simulink model "highgain_with_data_record_param_lowpass"  (R2021b)
settings: Solver=FixedStepDiscrete  StartTime=0.0  StopTime=10.0  RelTol=1e-3
values from neighbouring files (symbols this model uses):
  DEG2RAD = 0.0174533    [init.m]
  MAX_ATTI_INTEGRAL_SAT_LOWER = -1    [init.m]
  MAX_ATTI_INTEGRAL_SAT_UPPPER = 1    [init.m]
  MAX_ATTI_ROLLPITCH_CONTROL_COMMAND = 220 * DEG2RAD    (= 3.839726)    [init.m]
  MAX_ATTI_YAW_CONTROL_COMMAND = 200 * DEG2RAD    (= 3.49066)    [init.m]
  MAX_CONTROL_ANGLE_PITCH = 35    [init.m]
  MAX_CONTROL_ANGLE_RATE_Y = 200    [init.m]
  MAX_CONTROL_ANGLE_ROLL = 35    [init.m]
  MC_ROLL_P = Pixhawk_CSC.Parameter( {single(1), 'MC_ROLL_P'})    [init.m]
  MC_ROLLRATE_D = Pixhawk_CSC.Parameter( {single(1), 'MC_ROLLRATE_D'})    [init.m]
  MC_ROLLRATE_I = Pixhawk_CSC.Parameter( {single(1), 'MC_ROLLRATE_I'})    [init.m]
  MC_ROLLRATE_P = Pixhawk_CSC.Parameter( {single(1), 'MC_ROLLRATE_P'})    [init.m]
  THR_HOVER = 0.609    [init.m]
undefined symbols (not defined in the file or in its folder): DiscIntNeverNeededParam, RGBLED_COLOR_ENUM, RGBLED_MODE_ENUM
libraries: simulink x7, pixhawk_slib_sensors_actuators x5, pixhawk_slib_uORB_RW x4
settings Model: Creator=wsh  LastModifiedBy=jimdi
settings SolverCC: AlgebraicLoopSolver=TrustRegion
settings DataIOCC: ReturnWorkspaceOutputs=off
settings OptimizationCC: DefaultParameterBehavior=Inlined  MaxStackSize=64  EfficientTunableParamExpr=on
settings DebuggingCC: ParameterTunabilityLossMsg=error  SFMachineParentedDataDiag=warning  ArithmeticOperatorsInVariantConditions=warning
settings HardwareCC: ProdBitPerPointer=32  ProdBitPerSizeT=32  ProdBitPerPtrDiffT=32  ProdLargestAtomicInteger=Long  ProdLargestAtomicFloat=Double  ProdWordSize=32  ProdHWDeviceType=ARM Compatible->ARM Cortex
settings SFSimCC: SimUseLocalCustomCode=off  MATLABDynamicMemAlloc=off  CustomCodeUndefinedFunction=UseInterfaceOnly
settings RTWCC: Description=Embedded Coder  SystemTargetFile=ert.tlc  HardwareBoard=Pixhawk PX4  TLCOptions="-aInlineSetEventsForThisBaseRateFcn=TLC_FALSE -aSuppressMultiTaskScheduler=TLC_FALSE  -aRateBasedStepFcn=0"  TemplateMakefile=ert_default_tmf  GenerateReport=on  RTWUseLocalCustomCode=off  Toolchain=Pixhawk Toolchain  IncludeHyperlinkInReport=on  LaunchReport=on  GenerateTraceInfo=on  GenerateTraceReport=on  GenerateTraceReportSl=on  GenerateTraceReportSf=on  GenerateTraceReportEml=on
settings CodeAppCC: ForceParamTrailComments=on  IgnoreCustomStorageClasses=off  OperatorAnnotations=on  SimulinkDataObjDesc=on  SFDataObjDesc=on  MATLABFcnDesc=on  InsertBlockDesc=on  StateflowObjectComments=on  MATLABSourceComments=on
settings ERTTargetCC: MultiwordLength=2048  ERTCustomFileTemplate=PX4_codertarget_file_process.tlc

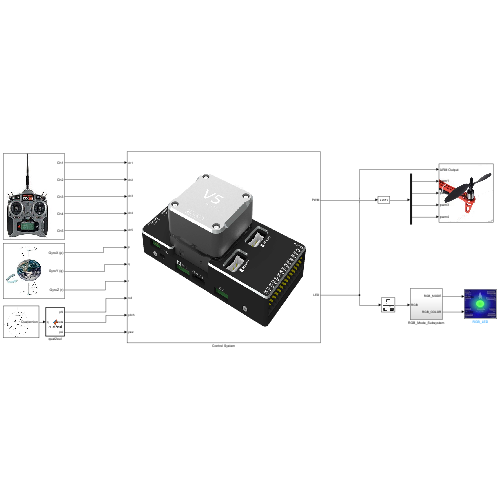
[thumbnail: Simulink's stored preview of the top-level diagram]
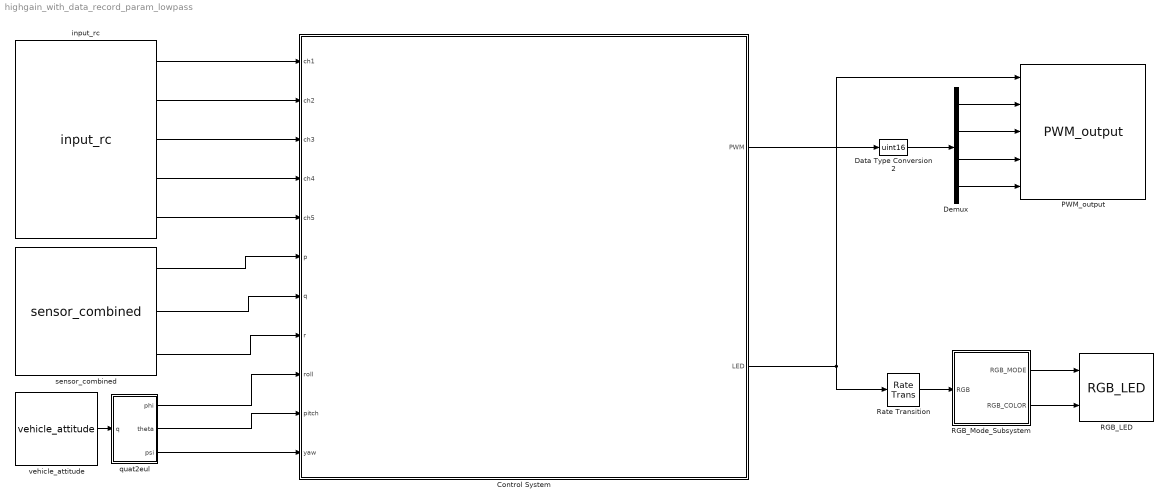
== system highgain_with_data_record_param_lowpass ==
  Control System : Subsystem
      mask Display: image('icon\pixhawk.png');
  Data Type Conversion2 : DataTypeConversion  OutDataTypeStr=uint16
  Demux : Demux
  PWM_output : pixhawk_slib_sensors_actuators/PWM_output  Description=|  pub_outputs=on  pwm_rate=400Hz  show_pwm1=on  show_pwm5=off  show_pwm2=on  show_pwm6=off  show_pwm3=on  show_pwm7=off  show_pwm4=on  show_pwm8=off
      | This block allows the user to send the appropriate PWM signals out to the PX4 outputs.  
      | These are usually connected to the ESCs which control the motor speeds. 
      | In order for the flight control to arm (enable) the output from the software side, the ARM Output input must be held high (boolean TRUE).  
      | Only then will the PWM values be sent out the PX4 hardware ports.  
      | This is usually a function of the RC Tx in combination with other flight modes programmed in the Simulink model by the user.  
      | The block has 8 available ports (data type uint16) which can be selectively chosen.  
      | These correspond to the 8 PWM output ports on the px4fmu hardware.
      settings: SourceProductName=Pixhawk Target Blocks
  RGB_LED : pixhawk_slib_sensors_actuators/RGB_LED
      settings: SourceProductName=Pixhawk Target Blocks
  RGB_Mode_Subsystem : Subsystem
  Rate Transition : RateTransition  OutPortSampleTime=1
  input_rc : pixhawk_slib_sensors_actuators/input_rc  Description=|  sampletime=0.004  channel1=on  channel2=on  channel3=on  channel4=on  channel5=on  channel6=off  channel7=off  channel8=off  channel9=off  channel10=off  channel11=off  channel12=off  channel13=off  channel14=off  channel15=off  channel16=off  channel17=off  channel18=off  ch_count=off  rssi=off  rc_failsafe=off  rc_lost=off  rc_inputsource=off
      | RC Input Block
      | 
      | This block provides user input control to the model.
      | It uses the input_rc uORB topic.
      | 
      | The user has the ability to choose which channels are available as outputs from this block and also some optional outputs. These include 
      | Channels 1 through 18
      | double data type indicating the PWM value from the controller 
      | measured pulse widths for each of the supported channels 
      | Channel Count 
      | uint32 data type of the number of channels which are detector by the PX4 
      | RC Failsafe 
      | boolean data types indicating that the RC Tx is sending the FailSafe signal (if equipped and properly setup) 
      | explicit failsafe flag: true on TX failure or TX out of range , false otherwise. 
      | Only the true state is reliable, as there are some (PPM) receivers on the market going into failsafe without telling us explicitly. 
      | RC Input Source 
      | Enumeration data type indicating which source the RC input is from. 
      | Valid values are found in the ENUM file: RC_INPUT_SOURCE_ENUM.m 
      |           Enumeration members for class 'RC_INPUT_SOURCE_ENUM':
      |           RCINPUT_SOURCE_UNKNOWN         (0)
      |           RCINPUT_SOURCE_PX4FMU_PPM      (1)
      |           RCINPUT_SOURCE_PX4IO_PPM       (2)
      |           RCINPUT_SOURCE_PX4IO_SPEKTRUM  (3)
      |           RCINPUT_SOURCE_PX4IO_SBUS      (4)
      |           RCINPUT_SOURCE_PX4IO_ST24      (5)
      |           RCINPUT_SOURCE_MAVLINK         (6)
      |           RCINPUT_SOURCE_QURT            (7)
      |           RCINPUT_SOURCE_PX4FMU_SPEKTRUM (8)
      |           RCINPUT_SOURCE_PX4FMU_SBUS     (9)
      |           RCINPUT_SOURCE_PX4FMU_ST24     (10)
      |           RCINPUT_SOURCE_PX4FMU_SUMD     (11)
      |           RCINPUT_SOURCE_PX4FMU_DSM      (12)
      |           RCINPUT_SOURCE_PX4IO_SUMD      (13)
      | 
      | RSSI - Receive signal strength index 
      | receive signal strength indicator (RSSI): < 0: Undefined, 0: no signal, 255: full reception 
      | RC Lost Connection 
      | boolean data type indicating RC receiver connection status 
      | True, if no frame has arrived in the expected time, false otherwise. 
      | True usally means that the receiver has been disconnected, but can also indicate a radio link loss on "stupid" systems. 
      | Will remain false, if a RX with failsafe option continues to transmit frames after a link loss. 
      |   
      | Sample Model: px4demo_input_rc.slx
      settings: SourceProductName=Pixhawk Target Blocks
  quat2eul : MATLAB Function  TreatAsAtomicUnit=on
  sensor_combined : pixhawk_slib_sensors_actuators/sensor_combined  Description=|  sampletime=0.004  show_mag=off  show_acc=off  show_gyro=on  show_baro=off  show_ts=off
      | Sensor Combined Block
      | 
      | This block enables access to the various sensors available on the px4fmu-v2 hardware.  
      | The user can use these signals in the Simulink control model.  
      | The sample time needs to be provided in the mask dialog.  
      | Optional output ports can also be selected.  
      | Refer to the sample model: px4demo_attitude_control.slx
      | 
      | Signal definitions: 
      | Magnetometer (x,y,z) - single values – Magnetic field in NED body frame, in Gauss 
      | Accelerometer (x,y,z) - single values – Acceleration in NED body frame, in m/s^2 
      | Gyroscope (p,q,r) - single values – Angular velocity in radians per second 
      | Barometer (Altitude) - single value – Barometric pressure, already temperature compensated (millibars) 
      | RunTime (timestamp) - double value – Timestamp in microseconds since boot, from gyro 
      |   
      | The sensor_combined block needs to have the px4io service running on the PX4 hardware in order to get valid signal values.
      settings: SourceProductName=Pixhawk Target Blocks
  vehicle_attitude : pixhawk_slib_sensors_actuators/vehicle_attitude  Description=|  sampletime=0.004  show_r=off  show_p=off  show_y=off  show_q=on  show_ts=off
      | This block gives access to the running service that calculates the vehicle’s attitude.  A uORB topic (vehicle_attitude (attitude measurements)) publisher MUST be running in order for this block to provide valid signal values.  The available ones as of v1.3 are: 
      | attitude_estimator_ekf – EKF-Extended Kalman Filter for attitude estimation 
      | attitude_estimator_so3 – SO(3)-attitude estimation by using accelerometer, gyroscopes and magnetometer 
      | One of these MUST be running on the px4fmu in order for this block to return valid values.  Refer to the sample model: px4demo_attitude_control.slx. Attitude in NED (North-East-Down) body frame in SI units. 
      | Signal definitions: 
      | Roll – single value, Roll angle (rad, Tait-Bryan, NED) 
      | Pitch – single value, Pitch angle (rad, Tait-Bryan, NED) 
      | Yaw – single value, Yaw angle (rad, Tait-Bryan, NED) 
      | Quaternion (NED) – single(4) values (optional based on the uORB publisher)
      settings: SourceProductName=Pixhawk Target Blocks
  wires:
  sensor_combined/1 -> Control System/6(p)
  sensor_combined/3 -> Control System/8(r)
  quat2eul/1(phi) -> Control System/9(roll)
  quat2eul/2(theta) -> Control System/10(pitch)
  sensor_combined/2 -> Control System/7(q)
  Control System/1(PWM) -> Data Type Conversion2/1
  Data Type Conversion2/1 -> Demux/1
  Demux/1 -> PWM_output/2
  Demux/2 -> PWM_output/3
  Demux/3 -> PWM_output/4
  Demux/4 -> PWM_output/5
  input_rc/1 -> Control System/1(ch1)
  input_rc/2 -> Control System/2(ch2)
  input_rc/3 -> Control System/3(ch3)
  input_rc/4 -> Control System/4(ch4)
  input_rc/5 -> Control System/5(ch5)
  RGB_Mode_Subsystem/2(RGB_COLOR) -> RGB_LED/2
  Rate Transition/1 -> RGB_Mode_Subsystem/1(RGB)
  RGB_Mode_Subsystem/1(RGB_MODE) -> RGB_LED/1
  Control System/2(LED) -> Rate Transition/1, PWM_output/1
  vehicle_attitude/1 -> quat2eul/1(q)
  quat2eul/3(psi) -> Control System/11(yaw)

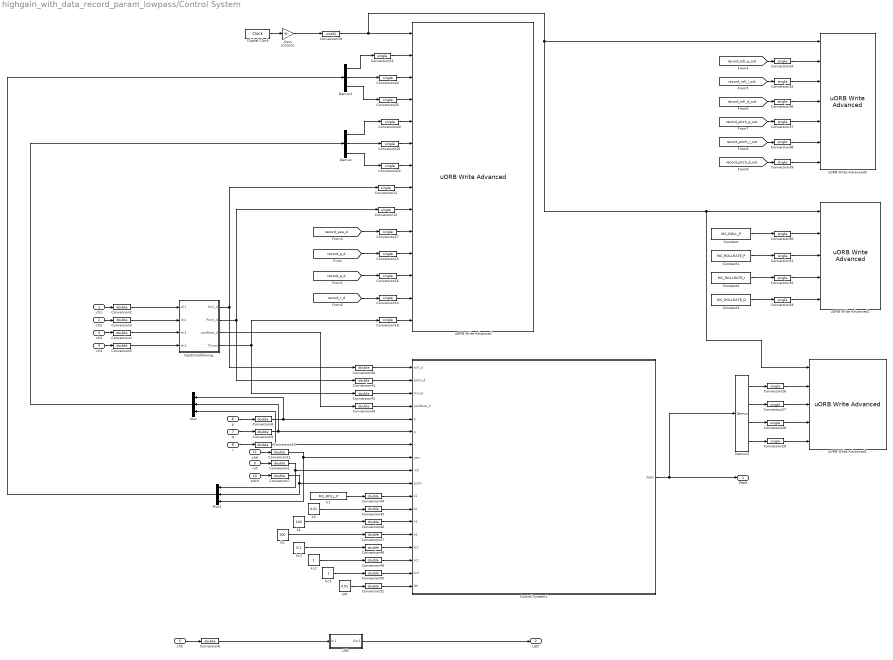
== system highgain_with_data_record_param_lowpass/Control System ==
  ch1 : Inport  OutDataTypeStr=uint16  PortDimensions=1
  ch2 : Inport  Port=2  OutDataTypeStr=uint16  PortDimensions=1
  ch3 : Inport  Port=3  OutDataTypeStr=uint16  PortDimensions=1
  ch4 : Inport  Port=4  OutDataTypeStr=uint16  PortDimensions=1
  ch5 : Inport  Port=5  OutDataTypeStr=uint16  PortDimensions=1  Interpolate=off
  p : Inport  Port=6  PortDimensions=1
  q : Inport  Port=7  PortDimensions=1
  r : Inport  Port=8  PortDimensions=1
  roll : Inport  Port=9  PortDimensions=1
  pitch : Inport  Port=10  PortDimensions=1
  yaw : Inport  Port=11  PortDimensions=1
  Constant : Constant  Value=MC_ROLL_P
  Constant1 : Constant  Value=MC_ROLLRATE_P
  Constant2 : Constant  Value=MC_ROLLRATE_I
  Constant3 : Constant  Value=MC_ROLLRATE_D
  Control System1 : Subsystem
      mask Display: image('test_bench.png'); % 使用工具条上的 "编辑图像" 进行更改。
  Conversion{1..11,40..51} (23 alike) : DataTypeConversion  OutDataTypeStr=double
  Conversion{12..18,20..39} (27 alike) : DataTypeConversion  OutDataTypeStr=single
  Conversion19 : DataTypeConversion  OutDataTypeStr=uint32
  Demux : Demux  Outputs=3
  Demux1 : Demux  Outputs=3
  Demux2 : Demux
  Digital Clock : DigitalClock  SampleTime=-1
  Gain : Gain  Gain=1000000
  InputConditioning : Subsystem
  "LED " : Subsystem
  Mux : Mux  Inputs=3
  Mux1 : Mux  Inputs=3
  h1 : Constant  Value=100
  h2 : Constant  Value=100
  k1 : Constant  Value=MC_ROLL_P
  k2 : Constant  Value=0.01
  kM : Constant  Value=0.01
  kc1 : Constant  Value=0.1
  kc2 : Constant
  kc3 : Constant
  uORB Write Advanced{,1..3} (4 alike) : pixhawk_slib_uORB_RW/uORB Write Advanced  Ts=0  uORB_AdvtQueue=on  uORB_FieldEnabledArr="0  0  0  1  0  0  0  0  0  0  0"  uORB_Topic_str=0  uORB_Struct_DT="[1  1  1  1  1]"  BlockInputCount=5  uORB_StructParams="[\"voltage_v\",\"voltage_filtered_v\",\"current_a\",\"current_filtered_a\",\"remaining\"]"  uORB_PortSizes="[1  1  1  1]"  MsgSizeOf=0  MW_update=true
      settings: SourceProductName=Pixhawk Target Blocks
  PWM : Outport  VectorParamsAs1DForOutWhenUnconnected=off
  LED : Outport  Port=2  PortDimensions=1  VectorParamsAs1DForOutWhenUnconnected=off
  wires:
  kc1/1 -> Conversion48/1
  Conversion9/1 -> Mux/2, Control System1/6(q)
  p/1 -> Conversion8/1
  "LED "/1(Out1) -> LED/1
  kM/1 -> Conversion51/1
  Conversion11/1 -> Mux1/3, Control System1/8(yaw)
  Control System1/1(PWM) -> Demux2/1, PWM/1
  Conversion4/1 -> InputConditioning/3(ch3)
  h2/1 -> Conversion47/1
  ch1/1 -> Conversion2/1
  h1/1 -> Conversion46/1
  ch4/1 -> Conversion5/1
  InputConditioning/4(Thrust) -> Conversion18/1, Conversion42/1
  Conversion2/1 -> InputConditioning/1("ch1 ")
  InputConditioning/3(yawRate_d) -> Conversion43/1
  Conversion1/1 -> Mux1/1, Control System1/9(roll)
  Conversion7/1 -> Mux1/2, Control System1/10(pitch)
  yaw/1 -> Conversion11/1
  kc3/1 -> Conversion50/1
  kc2/1 -> Conversion49/1
  Conversion8/1 -> Control System1/5(p), Mux/1
  InputConditioning/1(Roll_d) -> Conversion40/1, Conversion12/1
  Conversion10/1 -> Mux/3, Control System1/7(r)
  roll/1 -> Conversion1/1
  InputConditioning/2(Pitch_d) -> Conversion41/1, Conversion13/1
  k2/1 -> Conversion45/1
  Conversion3/1 -> InputConditioning/2(ch2)
  pitch/1 -> Conversion7/1
  r/1 -> Conversion10/1
  Conversion5/1 -> InputConditioning/4(ch4)
  Conversion6/1 -> "LED "/1(In1)
  ch2/1 -> Conversion3/1
  ch5/1 -> Conversion6/1
  ch3/1 -> Conversion4/1
  q/1 -> Conversion9/1
  Gain/1 -> Conversion19/1
  Conversion19/1 -> uORB Write Advanced2/1, uORB Write Advanced1/1, uORB Write Advanced3/1, uORB Write Advanced/1
  Digital Clock/1 -> Gain/1
  Conversion12/1 -> uORB Write Advanced/8
  Conversion13/1 -> uORB Write Advanced/9
  Mux/1 -> Demux/1
  Mux1/1 -> Demux1/1
  [record_p_d] -> Conversion15/1
  Conversion15/1 -> uORB Write Advanced/11
  Conversion16/1 -> uORB Write Advanced/12
  [record_q_d] -> Conversion16/1
  [record_r_d] -> Conversion14/1
  Conversion14/1 -> uORB Write Advanced/13
  [record_yaw_d] -> Conversion17/1
  Conversion17/1 -> uORB Write Advanced/10
  Conversion18/1 -> uORB Write Advanced/14
  Conversion20/1 -> uORB Write Advanced/5
  Conversion22/1 -> uORB Write Advanced/7
  Conversion21/1 -> uORB Write Advanced/6
  Demux/1 -> Conversion20/1
  Demux/2 -> Conversion21/1
  Demux/3 -> Conversion22/1
  Conversion25/1 -> uORB Write Advanced/4
  Conversion24/1 -> uORB Write Advanced/3
  Conversion23/1 -> uORB Write Advanced/2
  Demux1/1 -> Conversion23/1
  Demux1/2 -> Conversion24/1
  Demux1/3 -> Conversion25/1
  Conversion29/1 -> uORB Write Advanced1/5
  Conversion28/1 -> uORB Write Advanced1/4
  Conversion27/1 -> uORB Write Advanced1/3
  Conversion26/1 -> uORB Write Advanced1/2
  Demux2/1 -> Conversion26/1
  Demux2/2 -> Conversion27/1
  Demux2/3 -> Conversion28/1
  Demux2/4 -> Conversion29/1
  Conversion30/1 -> uORB Write Advanced2/2
  Conversion33/1 -> uORB Write Advanced2/5
  Conversion32/1 -> uORB Write Advanced2/4
  Conversion31/1 -> uORB Write Advanced2/3
  Constant/1 -> Conversion30/1
  Constant1/1 -> Conversion31/1
  Constant2/1 -> Conversion32/1
  Constant3/1 -> Conversion33/1
  Conversion34/1 -> uORB Write Advanced3/2
  [record_roll_p_out] -> Conversion34/1
  [record_roll_i_out] -> Conversion35/1
  Conversion35/1 -> uORB Write Advanced3/3
  Conversion36/1 -> uORB Write Advanced3/4
  [record_roll_d_out] -> Conversion36/1
  [record_pitch_p_out] -> Conversion37/1
  [record_pitch_i_out] -> Conversion38/1
  [record_pitch_d_out] -> Conversion39/1
  Conversion37/1 -> uORB Write Advanced3/5
  Conversion38/1 -> uORB Write Advanced3/6
  Conversion39/1 -> uORB Write Advanced3/7
  Conversion40/1 -> Control System1/1(roll_d)
  Conversion41/1 -> Control System1/2(pitch_d)
  Conversion42/1 -> Control System1/3(thrust)
  Conversion43/1 -> Control System1/4(yawRate_d)
  k1/1 -> Conversion44/1
  Conversion44/1 -> Control System1/11(k1)
  Conversion45/1 -> Control System1/12(k2)
  Conversion46/1 -> Control System1/13(h1)
  Conversion47/1 -> Control System1/14(h2)
  Conversion48/1 -> Control System1/15(kc1)
  Conversion49/1 -> Control System1/16(kc2)
  Conversion50/1 -> Control System1/17(kc3)
  Conversion51/1 -> Control System1/18(kM)

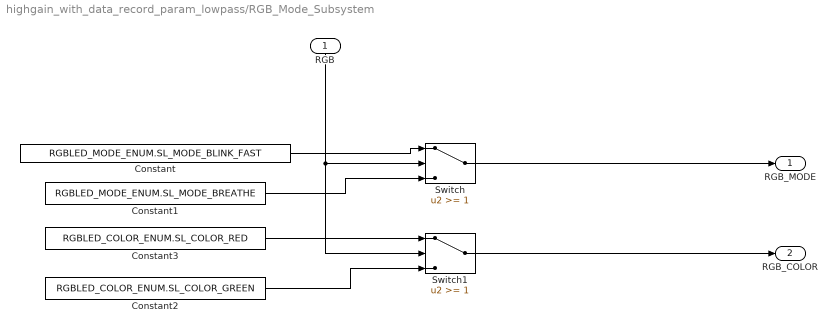
== system highgain_with_data_record_param_lowpass/RGB_Mode_Subsystem ==
  RGB : Inport
  Constant : Constant  Value=RGBLED_MODE_ENUM.SL_MODE_BLINK_FAST  OutDataTypeStr=Enum: RGBLED_MODE_ENUM
  Constant1 : Constant  Value=RGBLED_MODE_ENUM.SL_MODE_BREATHE  OutDataTypeStr=Enum: RGBLED_MODE_ENUM
  Constant2 : Constant  Value=RGBLED_COLOR_ENUM.SL_COLOR_GREEN  OutDataTypeStr=Enum: RGBLED_COLOR_ENUM
  Constant3 : Constant  Value=RGBLED_COLOR_ENUM.SL_COLOR_RED  OutDataTypeStr=Enum: RGBLED_COLOR_ENUM
  Switch : Switch  Threshold=1
  Switch1 : Switch  Threshold=1
  RGB_MODE : Outport  VectorParamsAs1DForOutWhenUnconnected=off
  RGB_COLOR : Outport  Port=2  VectorParamsAs1DForOutWhenUnconnected=off
  wires:
  RGB/1 -> Switch1/2, Switch/2
  Constant/1 -> Switch/1
  Constant1/1 -> Switch/3
  Switch/1 -> RGB_MODE/1
  Constant3/1 -> Switch1/1
  Constant2/1 -> Switch1/3
  Switch1/1 -> RGB_COLOR/1

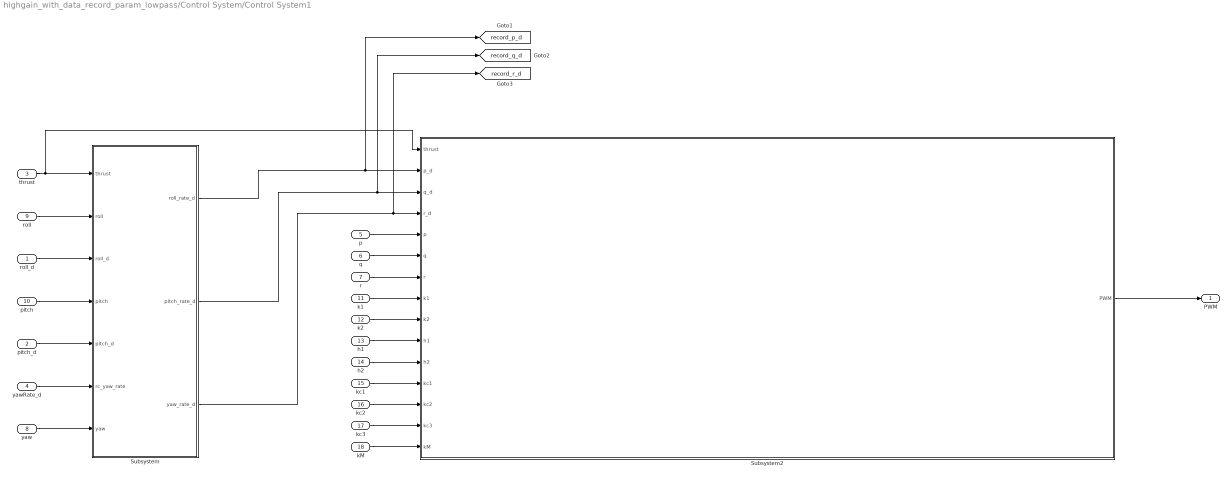
== system highgain_with_data_record_param_lowpass/Control System/Control System1 ==
  roll_d : Inport  PortDimensions=1
  pitch_d : Inport  Port=2  PortDimensions=1
  thrust : Inport  Port=3  PortDimensions=1
  yawRate_d : Inport  Port=4  PortDimensions=1
  p : Inport  Port=5  PortDimensions=1
  q : Inport  Port=6  PortDimensions=1
  r : Inport  Port=7  PortDimensions=1
  yaw : Inport  Port=8  PortDimensions=1
  roll : Inport  Port=9  PortDimensions=1
  pitch : Inport  Port=10  PortDimensions=1
  k1 : Inport  Port=11  PortDimensions=1
  k2 : Inport  Port=12  PortDimensions=1
  h1 : Inport  Port=13  PortDimensions=1
  h2 : Inport  Port=14  PortDimensions=1
  kc1 : Inport  Port=15  PortDimensions=1
  kc2 : Inport  Port=16  PortDimensions=1
  kc3 : Inport  Port=17  PortDimensions=1
  kM : Inport  Port=18  PortDimensions=1
  Subsystem : Subsystem
  Subsystem2 : Subsystem
      mask Display: image('angular_control_architecture.png'); % 使用工具条上的 "编辑图像" 进行更改。
  PWM : Outport  VectorParamsAs1DForOutWhenUnconnected=off
  tag scope: record_p_d=global, record_q_d=global, record_r_d=global
  wires:
  q/1 -> Subsystem2/6(q)
  r/1 -> Subsystem2/7(r)
  Subsystem2/1(PWM) -> PWM/1
  p/1 -> Subsystem2/5(p)
  k1/1 -> Subsystem2/8(k1)
  k2/1 -> Subsystem2/9(k2)
  h1/1 -> Subsystem2/10(h1)
  h2/1 -> Subsystem2/11(h2)
  kc1/1 -> Subsystem2/12(kc1)
  kc2/1 -> Subsystem2/13(kc2)
  kc3/1 -> Subsystem2/14(kc3)
  kM/1 -> Subsystem2/15(kM)
  thrust/1 -> Subsystem2/1(thrust), Subsystem/1(thrust)
  Subsystem/3(yaw_rate_d) -> [record_r_d], Subsystem2/4(r_d)
  Subsystem/2(pitch_rate_d) -> [record_q_d], Subsystem2/3(q_d)
  Subsystem/1(roll_rate_d) -> [record_p_d], Subsystem2/2(p_d)
  roll/1 -> Subsystem/2(roll)
  roll_d/1 -> Subsystem/3(roll_d)
  pitch/1 -> Subsystem/4(pitch)
  pitch_d/1 -> Subsystem/5(pitch_d)
  yawRate_d/1 -> Subsystem/6(rc_yaw_rate)
  yaw/1 -> Subsystem/7(yaw)

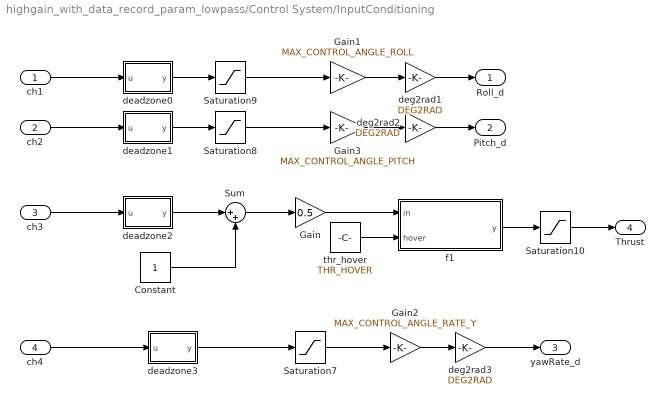
== system highgain_with_data_record_param_lowpass/Control System/InputConditioning ==
  "ch1 " : Inport
  ch2 : Inport  Port=2
  ch3 : Inport  Port=3
  ch4 : Inport  Port=4
  Constant : Constant
  Gain : Gain  Gain=0.5
  Gain1 : Gain  Gain=MAX_CONTROL_ANGLE_ROLL  OutDataTypeStr=Inherit: Inherit via back propagation
  Gain2 : Gain  Gain=MAX_CONTROL_ANGLE_RATE_Y
  Gain3 : Gain  Gain=MAX_CONTROL_ANGLE_PITCH  OutDataTypeStr=Inherit: Inherit via back propagation
  Saturation10 : Saturate  UpperLimit=1  LowerLimit=0
  Saturation7 : Saturate  UpperLimit=1  LowerLimit=-1
  Saturation8 : Saturate  UpperLimit=1  LowerLimit=-1
  Saturation9 : Saturate  UpperLimit=1  LowerLimit=-1
  Sum : Sum  Inputs=|++
  deadzone0 : MATLAB Function  TreatAsAtomicUnit=on
  deadzone1 : MATLAB Function  TreatAsAtomicUnit=on
  deadzone2 : MATLAB Function  TreatAsAtomicUnit=on
  deadzone3 : MATLAB Function  TreatAsAtomicUnit=on
  deg2rad1 : Gain  Gain=DEG2RAD
  deg2rad2 : Gain  Gain=DEG2RAD
  deg2rad3 : Gain  Gain=DEG2RAD
  f1 : MATLAB Function  TreatAsAtomicUnit=on
  "thr_hover " : Constant  Value=THR_HOVER
  Roll_d : Outport  VectorParamsAs1DForOutWhenUnconnected=off
  Pitch_d : Outport  Port=2  VectorParamsAs1DForOutWhenUnconnected=off
  yawRate_d : Outport  Port=3  VectorParamsAs1DForOutWhenUnconnected=off
  Thrust : Outport  Port=4  VectorParamsAs1DForOutWhenUnconnected=off
  wires:
  deadzone2/1(y) -> Sum/1
  ch3/1 -> deadzone2/1(u)
  deadzone1/1(y) -> Saturation8/1
  Saturation10/1 -> Thrust/1
  deadzone0/1(y) -> Saturation9/1
  "ch1 "/1 -> deadzone0/1(u)
  ch2/1 -> deadzone1/1(u)
  Saturation9/1 -> Gain1/1
  Saturation8/1 -> Gain3/1
  Gain3/1 -> deg2rad2/1
  Constant/1 -> Sum/2
  Sum/1 -> Gain/1
  Gain1/1 -> deg2rad1/1
  deg2rad1/1 -> Roll_d/1
  deg2rad2/1 -> Pitch_d/1
  Saturation7/1 -> Gain2/1
  deadzone3/1(y) -> Saturation7/1
  ch4/1 -> deadzone3/1(u)
  Gain2/1 -> deg2rad3/1
  deg2rad3/1 -> yawRate_d/1
  "thr_hover "/1 -> f1/2(hover)
  Gain/1 -> f1/1(in)
  f1/1(y) -> Saturation10/1

== system highgain_with_data_record_param_lowpass/Control System/LED  ==
  In1 : Inport
  Compare To Constant3 : simulink/Logic and Bit Operations/Compare To Constant  relop=>=  const=uint16(1500)  OutDataTypeStr=boolean
  Out1 : Outport  VectorParamsAs1DForOutWhenUnconnected=off
  wires:
  Compare To Constant3/1 -> Out1/1
  In1/1 -> Compare To Constant3/1

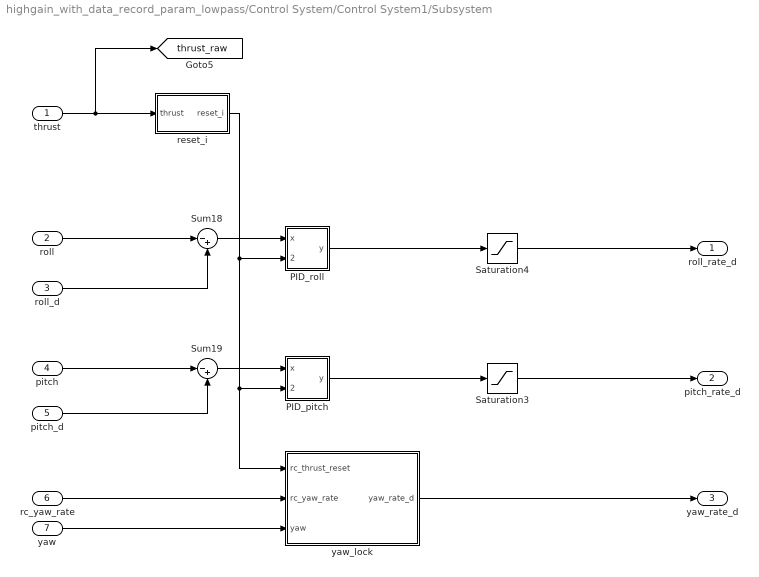
== system highgain_with_data_record_param_lowpass/Control System/Control System1/Subsystem ==
  thrust : Inport
  roll : Inport  Port=2
  roll_d : Inport  Port=3
  pitch : Inport  Port=4
  pitch_d : Inport  Port=5
  rc_yaw_rate : Inport  Port=6
  yaw : Inport  Port=7
  PID_pitch : Subsystem
  "PID_roll " : Subsystem
  Saturation3 : Saturate  UpperLimit=MAX_ATTI_ROLLPITCH_CONTROL_COMMAND  LowerLimit=-MAX_ATTI_ROLLPITCH_CONTROL_COMMAND
  Saturation4 : Saturate  UpperLimit=MAX_ATTI_ROLLPITCH_CONTROL_COMMAND  LowerLimit=-MAX_ATTI_ROLLPITCH_CONTROL_COMMAND
  Sum18 : Sum  Inputs=|-+
  Sum19 : Sum  Inputs=|-+
  reset_i : Subsystem
  yaw_lock : Subsystem
  roll_rate_d : Outport
  pitch_rate_d : Outport  Port=2
  yaw_rate_d : Outport  Port=3
  tag scope: thrust_raw=global
  wires:
  "PID_roll "/1(y) -> Saturation4/1
  reset_i/1(reset_i) -> yaw_lock/1(rc_thrust_reset), PID_pitch/2(reset_i), "PID_roll "/2(reset_i)
  pitch/1 -> Sum19/1
  Sum19/1 -> PID_pitch/1(x)
  PID_pitch/1(y) -> Saturation3/1
  Sum18/1 -> "PID_roll "/1(x)
  yaw/1 -> yaw_lock/3(yaw)
  roll/1 -> Sum18/1
  yaw_lock/1(yaw_rate_d) -> yaw_rate_d/1
  rc_yaw_rate/1 -> yaw_lock/2(rc_yaw_rate)
  pitch_d/1 -> Sum19/2
  roll_d/1 -> Sum18/2
  Saturation3/1 -> pitch_rate_d/1
  Saturation4/1 -> roll_rate_d/1
  thrust/1 -> [thrust_raw], reset_i/1(thrust)

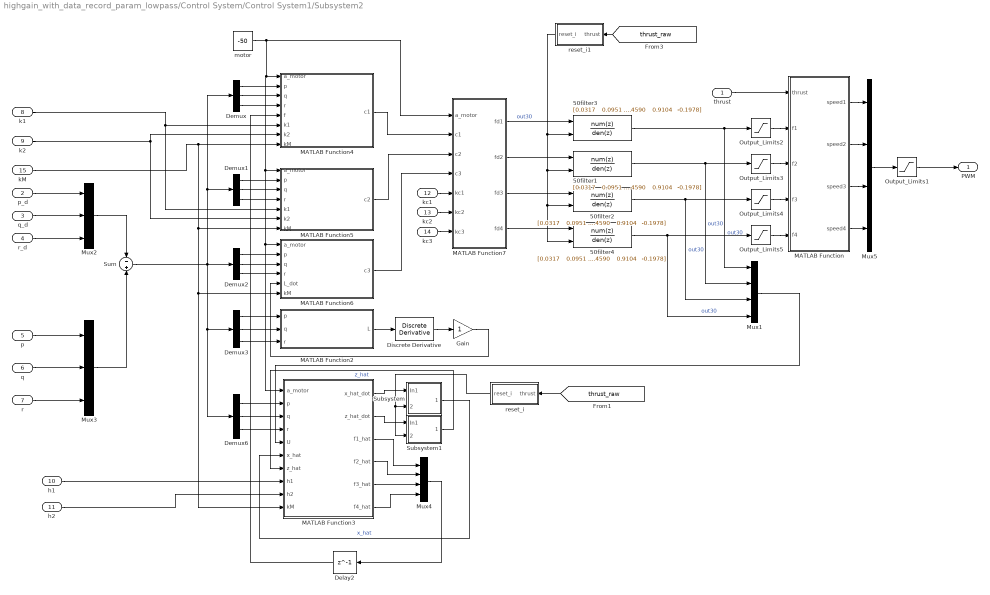
== system highgain_with_data_record_param_lowpass/Control System/Control System1/Subsystem2 ==
  thrust : Inport
  p_d : Inport  Port=2  PortDimensions=1
  q_d : Inport  Port=3  PortDimensions=1
  r_d : Inport  Port=4  PortDimensions=1
  p : Inport  Port=5  PortDimensions=1
  q : Inport  Port=6  PortDimensions=1
  r : Inport  Port=7  PortDimensions=1
  k1 : Inport  Port=8  PortDimensions=1
  k2 : Inport  Port=9  PortDimensions=1
  h1 : Inport  Port=10  PortDimensions=1
  h2 : Inport  Port=11  PortDimensions=1
  kc1 : Inport  Port=12  PortDimensions=1
  kc2 : Inport  Port=13  PortDimensions=1
  kc3 : Inport  Port=14  PortDimensions=1
  kM : Inport  Port=15  PortDimensions=1
  50filter{1..4} (4 alike) : DiscreteFilter  Numerator="[0.0317    0.0951    0.0951    0.0317]"  Denominator="[1.0000   -1.4590    0.9104   -0.1978]"  ExternalReset=Level
      settings: InputPortMap=u0,r7
  Delay2 : Delay  DelayLength=1  InitialCondition=0  SampleTime=0.001
  Demux{,1..3,6} (5 alike) : Demux  Outputs=3
  Discrete Derivative : simulink/Discrete/Discrete Derivative  gainval=1.0  ICPrevScaledInput=0.0  OutMin=[]  OutMax=[]  OutDataType=fixdt(1, 16)  OutScaling=2^-10  DoSatur=off
  Gain : Gain
  MATLAB Function : MATLAB Function  TreatAsAtomicUnit=on
  MATLAB Function2 : MATLAB Function  TreatAsAtomicUnit=on
  MATLAB Function3 : MATLAB Function  TreatAsAtomicUnit=on
  MATLAB Function4 : MATLAB Function  TreatAsAtomicUnit=on
  MATLAB Function5 : MATLAB Function  TreatAsAtomicUnit=on
  MATLAB Function6 : MATLAB Function  TreatAsAtomicUnit=on
  MATLAB Function7 : MATLAB Function  TreatAsAtomicUnit=on
  Mux1 : Mux
  Mux2 : Mux  Inputs=3
  Mux3 : Mux  Inputs=3
  Mux4 : Mux
  Mux5 : Mux
  Output_Limits1 : Saturate  UpperLimit=1950  LowerLimit=1230  LinearizeAsGain=off
  Output_Limits{2..5} (4 alike) : Saturate  UpperLimit=1  LowerLimit=-1  LinearizeAsGain=off
  Subsystem : Subsystem
  Subsystem1 : Subsystem
  Sum : Sum  Inputs=-+
  motor : Constant  Value=-50
  reset_i : Subsystem
  reset_i1 : Subsystem
  PWM : Outport
  wires:
  Demux/3 -> MATLAB Function4/4(r)
  Mux2/1 -> Sum/1
  MATLAB Function/2(speed2) -> Mux5/2
  Subsystem1/1(Out1) -> MATLAB Function3/7(z_hat)  "z_hat"
  Demux3/1 -> MATLAB Function2/1(p)
  MATLAB Function3/3(f1_hat) -> Mux4/1
  MATLAB Function5/1(c2) -> MATLAB Function7/3(c2)
  Demux6/1 -> MATLAB Function3/2(p)
  Mux4/1 -> Delay2/1
  k2/1 -> MATLAB Function4/7(k2), MATLAB Function5/6(k2)
  q_d/1 -> Mux2/2
  MATLAB Function/1(speed1) -> Mux5/1
  Demux2/2 -> MATLAB Function6/3(q)
  Demux3/2 -> MATLAB Function2/2(q)
  Demux6/3 -> MATLAB Function3/4(r)
  Demux/2 -> MATLAB Function4/3(q)
  Demux/1 -> MATLAB Function4/2(p)
  MATLAB Function3/5(f3_hat) -> Mux4/3
  MATLAB Function3/6(f4_hat) -> Mux4/4
  Gain/1 -> MATLAB Function6/5(L_dot)
  motor/1 -> MATLAB Function7/1(a_motor), MATLAB Function3/1(a_motor), MATLAB Function6/1(a_motor), MATLAB Function5/1(a_motor), MATLAB Function4/1(a_motor)
  MATLAB Function/3(speed3) -> Mux5/3
  MATLAB Function6/1(c3) -> MATLAB Function7/4(c3)
  Subsystem/1(Out1) -> MATLAB Function3/6(x_hat)  "x_hat"
  Demux2/1 -> MATLAB Function6/2(p)
  Demux1/1 -> MATLAB Function5/2(p)
  MATLAB Function3/1(x_hat_dot) -> Subsystem/1(In1)
  Demux3/3 -> MATLAB Function2/3(r)
  Demux6/2 -> MATLAB Function3/3(q)
  MATLAB Function3/2(z_hat_dot) -> Subsystem1/1(In1)
  Sum/1 -> Demux6/1, Demux3/1, Demux/1, Demux1/1, Demux2/1
  MATLAB Function4/1(c1) -> MATLAB Function7/2(c1)
  Demux2/3 -> MATLAB Function6/4(r)
  r_d/1 -> Mux2/3
  Output_Limits1/1 -> PWM/1
  Demux1/3 -> MATLAB Function5/4(r)
  p_d/1 -> Mux2/1
  thrust/1 -> MATLAB Function/1(thrust)
  Mux5/1 -> Output_Limits1/1
  MATLAB Function3/4(f2_hat) -> Mux4/2
  k1/1 -> MATLAB Function5/5(k1), MATLAB Function4/6(k1)
  MATLAB Function2/1(L) -> Discrete Derivative/1
  Demux1/2 -> MATLAB Function5/3(q)
  MATLAB Function/4(speed4) -> Mux5/4
  Delay2/1 -> MATLAB Function4/5(f)
  Output_Limits2/1 -> MATLAB Function/2(f1)
  Output_Limits3/1 -> MATLAB Function/3(f2)
  Output_Limits4/1 -> MATLAB Function/4(f3)
  Output_Limits5/1 -> MATLAB Function/5(f4)
  h1/1 -> MATLAB Function3/8(h1)
  h2/1 -> MATLAB Function3/9(h2)
  kc1/1 -> MATLAB Function7/5(kc1)
  kc2/1 -> MATLAB Function7/6(kc2)
  kc3/1 -> MATLAB Function7/7(kc3)
  kM/1 -> MATLAB Function3/10(kM), MATLAB Function6/6(kM), MATLAB Function5/7(kM), MATLAB Function4/8(kM)
  Discrete Derivative/1 -> Gain/1
  Mux1/1 -> MATLAB Function3/5(U)
  Mux3/1 -> Sum/2
  MATLAB Function7/1(fd1) -> 50filter3/1  "out30"
  50filter3/1 -> Mux1/1, Output_Limits2/1  "out30"
  MATLAB Function7/2(fd2) -> 50filter1/1
  50filter1/1 -> Mux1/2, Output_Limits3/1  "out30"
  MATLAB Function7/3(fd3) -> 50filter2/1
  50filter2/1 -> Mux1/3, Output_Limits4/1  "out30"
  MATLAB Function7/4(fd4) -> 50filter4/1
  50filter4/1 -> Output_Limits5/1, Mux1/4  "out30"
  reset_i1/1(reset_i) -> 50filter3/2, 50filter1/2, 50filter4/2, 50filter2/2
  p/1 -> Mux3/1
  q/1 -> Mux3/2
  r/1 -> Mux3/3
  [thrust_raw] -> reset_i/1(thrust)
  reset_i/1(reset_i) -> Subsystem1/2(reset), Subsystem/2(reset)
  [thrust_raw] -> reset_i1/1(thrust)

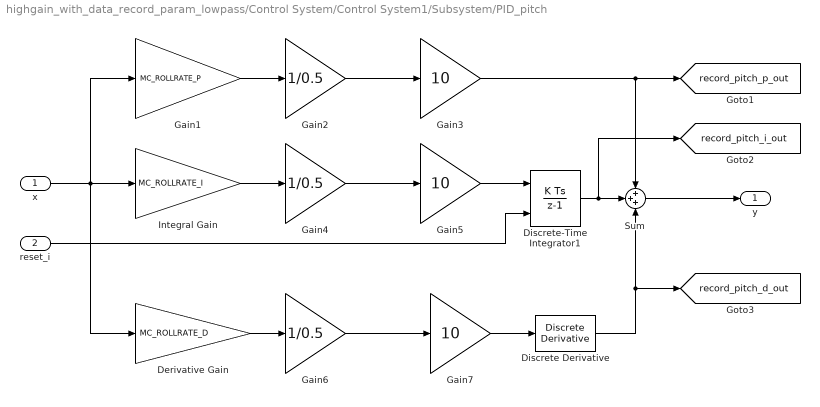
== system highgain_with_data_record_param_lowpass/Control System/Control System1/Subsystem/PID_pitch ==
  x : Inport
  reset_i : Inport  Port=2
  Derivative Gain : Gain  DisableCoverage=on  Gain=MC_ROLLRATE_D  ParamMin=-100  ParamMax=100  OutMin=-100  OutMax=100
  Discrete Derivative : simulink/Discrete/Discrete Derivative  gainval=1.0  ICPrevScaledInput=0.0  OutMin=[]  OutMax=[]  OutDataType=fixdt(1, 16)  OutScaling=2^-10  DoSatur=off
  Discrete-Time Integrator1 : DiscreteIntegrator  ExternalReset=level  SampleTime=-1  LimitOutput=on  UpperSaturationLimit=MAX_ATTI_INTEGRAL_SAT_UPPPER  LowerSaturationLimit=MAX_ATTI_INTEGRAL_SAT_LOWER  ICPrevOutput=DiscIntNeverNeededParam  ICPrevScaledInput=DiscIntNeverNeededParam
  Gain1 : Gain  Gain=MC_ROLLRATE_P
  Gain2 : Gain  Gain=1/0.5
  Gain3 : Gain  Gain=10
  Gain4 : Gain  Gain=1/0.5
  Gain5 : Gain  Gain=10
  Gain6 : Gain  Gain=1/0.5
  Gain7 : Gain  Gain=10
  Integral Gain : Gain  DisableCoverage=on  Gain=MC_ROLLRATE_I
  Sum : Sum  Inputs=+++
  y : Outport  InitialOutput=0  VectorParamsAs1DForOutWhenUnconnected=off
  tag scope: record_pitch_d_out=global, record_pitch_i_out=global, record_pitch_p_out=global
  wires:
  reset_i/1 -> Discrete-Time Integrator1/2
  Discrete Derivative/1 -> Sum/3, [record_pitch_d_out]
  Sum/1 -> y/1
  x/1 -> Derivative Gain/1, Integral Gain/1, Gain1/1
  Discrete-Time Integrator1/1 -> [record_pitch_i_out], Sum/2
  Gain1/1 -> Gain2/1
  Gain2/1 -> Gain3/1
  Gain3/1 -> [record_pitch_p_out], Sum/1
  Gain5/1 -> Discrete-Time Integrator1/1
  Gain4/1 -> Gain5/1
  Integral Gain/1 -> Gain4/1
  Derivative Gain/1 -> Gain6/1
  Gain7/1 -> Discrete Derivative/1
  Gain6/1 -> Gain7/1

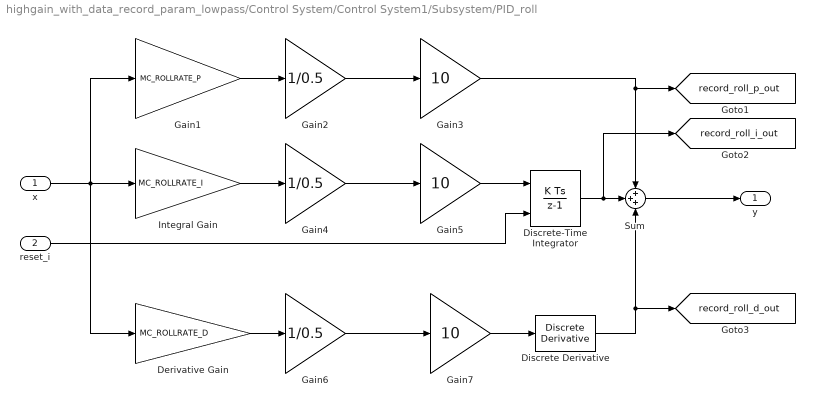
== system highgain_with_data_record_param_lowpass/Control System/Control System1/Subsystem/PID_roll  ==
  x : Inport
  reset_i : Inport  Port=2
  Derivative Gain : Gain  DisableCoverage=on  Gain=MC_ROLLRATE_D  ParamMin=-100  ParamMax=100  OutMin=-100  OutMax=100
  Discrete Derivative : simulink/Discrete/Discrete Derivative  gainval=1.0  ICPrevScaledInput=0.0  OutMin=[]  OutMax=[]  OutDataType=fixdt(1, 16)  OutScaling=2^-10  DoSatur=off
  Discrete-Time Integrator : DiscreteIntegrator  ExternalReset=level  SampleTime=-1  LimitOutput=on  UpperSaturationLimit=MAX_ATTI_INTEGRAL_SAT_UPPPER  LowerSaturationLimit=MAX_ATTI_INTEGRAL_SAT_LOWER  ICPrevOutput=DiscIntNeverNeededParam  ICPrevScaledInput=DiscIntNeverNeededParam
  Gain1 : Gain  Gain=MC_ROLLRATE_P
  Gain2 : Gain  Gain=1/0.5
  Gain3 : Gain  Gain=10
  Gain4 : Gain  Gain=1/0.5
  Gain5 : Gain  Gain=10
  Gain6 : Gain  Gain=1/0.5
  Gain7 : Gain  Gain=10
  Integral Gain : Gain  DisableCoverage=on  Gain=MC_ROLLRATE_I
  Sum : Sum  Inputs=+++
  y : Outport  InitialOutput=0  VectorParamsAs1DForOutWhenUnconnected=off
  tag scope: record_roll_d_out=global, record_roll_i_out=global, record_roll_p_out=global
  wires:
  reset_i/1 -> Discrete-Time Integrator/2
  Discrete Derivative/1 -> [record_roll_d_out], Sum/3
  Sum/1 -> y/1
  x/1 -> Derivative Gain/1, Integral Gain/1, Gain1/1
  Discrete-Time Integrator/1 -> [record_roll_i_out], Sum/2
  Gain1/1 -> Gain2/1
  Gain2/1 -> Gain3/1
  Gain3/1 -> Sum/1, [record_roll_p_out]
  Gain5/1 -> Discrete-Time Integrator/1
  Gain4/1 -> Gain5/1
  Integral Gain/1 -> Gain4/1
  Derivative Gain/1 -> Gain6/1
  Gain7/1 -> Discrete Derivative/1
  Gain6/1 -> Gain7/1

== system highgain_with_data_record_param_lowpass/Control System/Control System1/Subsystem/reset_i ==
  thrust : Inport
  Compare To Constant3 : simulink/Logic and Bit Operations/Compare To Constant  relop=<=  const=0.3  OutDataTypeStr=boolean
  reset_i : Outport  VectorParamsAs1DForOutWhenUnconnected=off
  wires:
  thrust/1 -> Compare To Constant3/1
  Compare To Constant3/1 -> reset_i/1

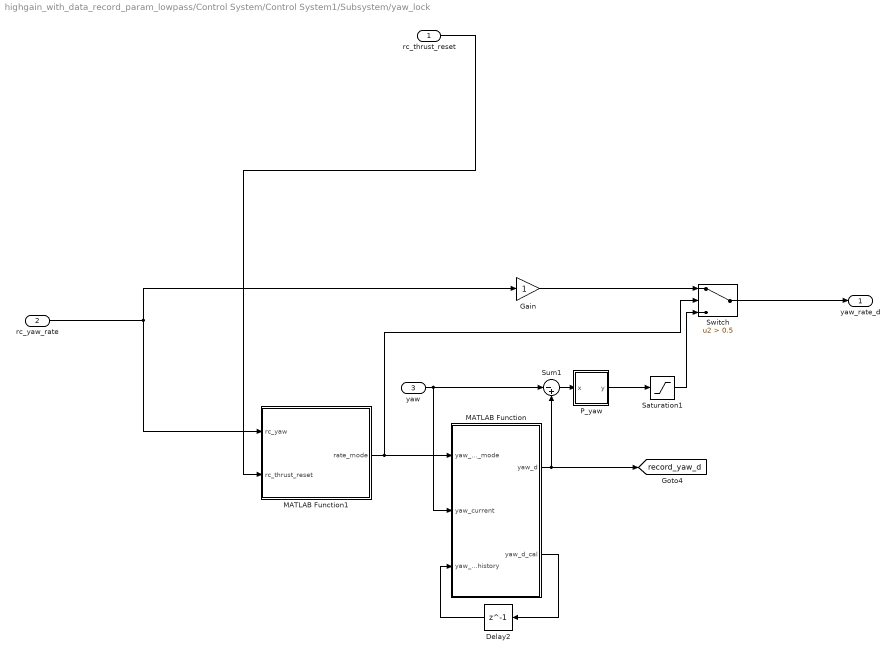
== system highgain_with_data_record_param_lowpass/Control System/Control System1/Subsystem/yaw_lock ==
  rc_thrust_reset : Inport
  rc_yaw_rate : Inport  Port=2
  yaw : Inport  Port=3  PortDimensions=1
  Delay2 : Delay  DelayLength=1  InitialCondition=0  SampleTime=0.001
  Gain : Gain
  MATLAB Function : MATLAB Function  TreatAsAtomicUnit=on
  MATLAB Function1 : MATLAB Function  TreatAsAtomicUnit=on
  P_yaw : Subsystem
  Saturation1 : Saturate  UpperLimit=MAX_ATTI_YAW_CONTROL_COMMAND  LowerLimit=-MAX_ATTI_YAW_CONTROL_COMMAND
  Sum1 : Sum  Inputs=|-+
  Switch : Switch  Criteria=u2 > Threshold  Threshold=0.5
  yaw_rate_d : Outport
  tag scope: record_yaw_d=global
  wires:
  rc_yaw_rate/1 -> Gain/1, MATLAB Function1/1(rc_yaw)
  Saturation1/1 -> Switch/3
  P_yaw/1(y) -> Saturation1/1
  Sum1/1 -> P_yaw/1(x)
  MATLAB Function1/1(rate_mode) -> Switch/2, MATLAB Function/1(yaw_rate_mode)
  MATLAB Function/2(yaw_d_cal) -> Delay2/1
  MATLAB Function/1(yaw_d) -> [record_yaw_d], Sum1/2
  Delay2/1 -> MATLAB Function/3(yaw_d_history)
  Gain/1 -> Switch/1
  yaw/1 -> Sum1/1, MATLAB Function/2(yaw_current)
  rc_thrust_reset/1 -> MATLAB Function1/2(rc_thrust_reset)
  Switch/1 -> yaw_rate_d/1

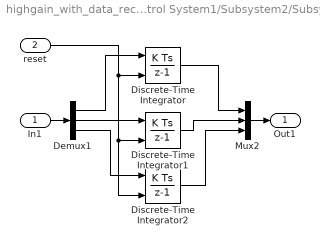
== system highgain_with_data_record_param_lowpass/Control System/Control System1/Subsystem2/Subsystem ==
  In1 : Inport
  reset : Inport  Port=2
  Demux1 : Demux  Outputs=3
  Discrete-Time Integrator : DiscreteIntegrator  ExternalReset=level  SampleTime=-1  OutDataTypeStr=double  ICPrevOutput=DiscIntNeverNeededParam  ICPrevScaledInput=DiscIntNeverNeededParam
  Discrete-Time Integrator1 : DiscreteIntegrator  ExternalReset=level  SampleTime=-1  OutDataTypeStr=double  ICPrevOutput=DiscIntNeverNeededParam  ICPrevScaledInput=DiscIntNeverNeededParam
  Discrete-Time Integrator2 : DiscreteIntegrator  ExternalReset=level  SampleTime=-1  OutDataTypeStr=double  ICPrevOutput=DiscIntNeverNeededParam  ICPrevScaledInput=DiscIntNeverNeededParam
  Mux2 : Mux  Inputs=3
  Out1 : Outport
  wires:
  Discrete-Time Integrator2/1 -> Mux2/3
  Demux1/2 -> Discrete-Time Integrator1/1
  Demux1/3 -> Discrete-Time Integrator2/1
  Discrete-Time Integrator/1 -> Mux2/1
  Demux1/1 -> Discrete-Time Integrator/1
  In1/1 -> Demux1/1
  Mux2/1 -> Out1/1
  Discrete-Time Integrator1/1 -> Mux2/2
  reset/1 -> Discrete-Time Integrator/2, Discrete-Time Integrator2/2, Discrete-Time Integrator1/2

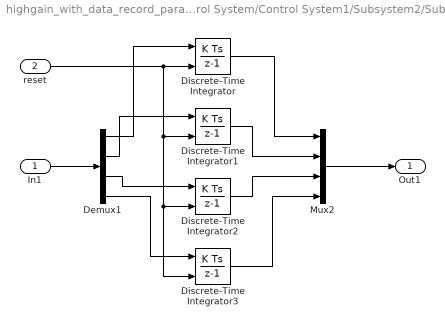
== system highgain_with_data_record_param_lowpass/Control System/Control System1/Subsystem2/Subsystem1 ==
  In1 : Inport
  reset : Inport  Port=2
  Demux1 : Demux
  Discrete-Time Integrator{,1..3} (4 alike) : DiscreteIntegrator  ExternalReset=level  SampleTime=-1  OutDataTypeStr=double  ICPrevOutput=DiscIntNeverNeededParam  ICPrevScaledInput=DiscIntNeverNeededParam
  Mux2 : Mux
  Out1 : Outport
  wires:
  Discrete-Time Integrator/1 -> Mux2/1
  In1/1 -> Demux1/1
  Mux2/1 -> Out1/1
  Demux1/1 -> Discrete-Time Integrator/1
  Demux1/2 -> Discrete-Time Integrator1/1
  Discrete-Time Integrator1/1 -> Mux2/2
  Demux1/3 -> Discrete-Time Integrator2/1
  Discrete-Time Integrator2/1 -> Mux2/3
  Demux1/4 -> Discrete-Time Integrator3/1
  Discrete-Time Integrator3/1 -> Mux2/4
  reset/1 -> Discrete-Time Integrator3/2, Discrete-Time Integrator2/2, Discrete-Time Integrator1/2, Discrete-Time Integrator/2

== system highgain_with_data_record_param_lowpass/Control System/Control System1/Subsystem2/reset_i ==
  thrust : Inport
  Compare To Constant3 : simulink/Logic and Bit Operations/Compare To Constant  relop=<=  const=0.2  OutDataTypeStr=boolean
  reset_i : Outport  VectorParamsAs1DForOutWhenUnconnected=off
  wires:
  thrust/1 -> Compare To Constant3/1
  Compare To Constant3/1 -> reset_i/1

== system highgain_with_data_record_param_lowpass/Control System/Control System1/Subsystem2/reset_i1 ==
  thrust : Inport
  Compare To Constant3 : simulink/Logic and Bit Operations/Compare To Constant  relop=<=  const=0.1  OutDataTypeStr=boolean
  reset_i : Outport  VectorParamsAs1DForOutWhenUnconnected=off
  wires:
  thrust/1 -> Compare To Constant3/1
  Compare To Constant3/1 -> reset_i/1

== system highgain_with_data_record_param_lowpass/Control System/Control System1/Subsystem/yaw_lock/P_yaw ==
  x : Inport
  Gain : Gain  Gain=5.0119
  y : Outport  InitialOutput=0  VectorParamsAs1DForOutWhenUnconnected=off
  wires:
  x/1 -> Gain/1
  Gain/1 -> y/1

== matlab function highgain_with_data_record_param_lowpass/Control System/Control System1/Subsystem2/MATLAB Function3 ==
  data: a_motor input; p input; q input; r input; U input; x_hat input; x_hat_dot output; z_hat_dot output; z_hat input; f1_hat output; f2_hat output; f3_hat output; f4_hat output; h1 input; h2 input; kM input
function [x_hat_dot, z_hat_dot, f1_hat, f2_hat, f3_hat, f4_hat] = fcn(a_motor, p,q,r, U, x_hat, z_hat, h1, h2, kM)
I_xx = 0.0211;I_yy = 0.0211;I_zz = 0.0366;
L = [(1/I_xx) * (q * r * (I_yy - I_zz) );
     (1/I_yy) * (p * r * (I_zz - I_xx) );
     (1/I_zz) * (p * q * (I_xx - I_yy) )];
M_inv = kM*[-1,  1,  1;
          1, -1,  1;
          1,  1, -1;
         -1, -1, -1];
M = kM*0.25 * [-1,  1,  1, -1;
             1, -1,  1, -1;
             1,  1, -1, -1];
a = a_motor;
b = -a;
y = [p;q;r];
x_hat_dot = L       + M*z_hat   + h1*(y-x_hat);
z_hat_dot = a*z_hat + b*U       + h2*M_inv*(y-x_hat);
f1_hat = z_hat(1);
f2_hat = z_hat(2);
f3_hat = z_hat(3);
f4_hat = z_hat(4);
end

== matlab function highgain_with_data_record_param_lowpass/Control System/Control System1/Subsystem2/MATLAB Function4 ==
  data: a_motor input; p input; c1 output; q input; r input; f input; k1 input; k2 input; kM input
function c1 = C1_FCN(a_motor, p,q,r,f,k1,k2, kM)
A = a_motor * eye(4);
I = eye(4);
M_inv = kM*[-1,  1,  1;
          1, -1,  1;
          1,  1, -1;
         -1, -1, -1];
I_xx = 0.0211;I_yy = 0.0211;I_zz = 0.0366;
L = [q * r * (I_yy - I_zz);
     p * r * (I_zz - I_xx);
     p * q * (I_xx - I_yy)];
x = [p;q;r];
fan = -M_inv*(L+k1*x);
enta = f - fan;
c1 = -(A + k1*I + k2*I)*enta;
end

== matlab function highgain_with_data_record_param_lowpass/Control System/Control System1/Subsystem2/MATLAB Function5 ==
  data: a_motor input; p input; c2 output; q input; r input; k1 input; k2 input; kM input
function c2 = C2_FCN(a_motor, p,q, r,k1,k2,kM)
A = a_motor * eye(4);
M_inv = kM*[-1,  1,  1;
          1, -1,  1;
          1,  1, -1;
         -1, -1, -1];
M = kM*0.25 * [-1,  1,  1, -1;
             1, -1,  1, -1;
             1,  1, -1, -1];
epislo = [p;q;r];
c2 = (A*k1*M_inv + k1*k1*M_inv - M')*epislo;
end

== matlab function highgain_with_data_record_param_lowpass/Control System/Control System1/Subsystem2/MATLAB Function6 ==
  data: a_motor input; p input; c3 output; q input; r input; L_dot input; kM input
function c3 = C3_FCN(a_motor, p,q,r,L_dot, kM)
A = a_motor * eye(4);
M_inv = kM*[-1,  1,  1;
          1, -1,  1;
          1,  1, -1;
         -1, -1, -1];
I_xx = 0.0211;I_yy = 0.0211;I_zz = 0.0366;
L = [q * r * (I_yy - I_zz);
     p * r * (I_zz - I_xx);
     p * q * (I_xx - I_yy)];
%% need m dot
c3=A*M_inv*L - M_inv*L_dot;
end

== matlab function highgain_with_data_record_param_lowpass/Control System/Control System1/Subsystem2/MATLAB Function7 ==
  data: a_motor input; c1 input; fd1 output; fd2 output; fd3 output; fd4 output; c2 input; c3 input; kc1 input; kc2 input; kc3 input
function [fd1, fd2, fd3, fd4] = fcn(a_motor, c1, c2, c3, kc1, kc2, kc3)
b = -a_motor;
temp = kc1*c1 + kc2*c2 + kc3*c3;
temp = (1/b) * temp;
fd1 = temp(1);
fd2 = temp(2);
fd3 = temp(3);
fd4 = temp(4);
end

== matlab function highgain_with_data_record_param_lowpass/Control System/InputConditioning/f1 ==
  data: in input; y output; hover input
function y = thr_curve(in, hover)
%Function description:
%  After this function, when the throttle is in the middle position, the output is hovering throttle hover
%Input:
%  in: Throttle normalized value, range (0~1)
%  hover: Hovering throttle value
%Output:
%  Processed throttle value
if in < 0.5
	y=2 * in * hover;
else
	y=hover + 2 * (in - 0.5) * (1.0 - hover);
end

== matlab function highgain_with_data_record_param_lowpass/Control System/InputConditioning/deadzone0 ==
  data: u input; y output
function y = fcn(u)
%Function description:
%  Control the range of the remote control input from RCMin to RCMax, and set
%  a dead zone with a dead zone size of ±deadZone,the output y is
%  normalized to 0~1.You can get the RC calibration parameters in QGC.
RCMin = 1065;
RCMax = 1932;
RCMid = (RCMin + RCMax)/2;
deadZoneRate = 0.05;
deadZone = deadZoneRate*(RCMax - RCMin);
k = 1/(RCMax - RCMid - deadZone);
%Limiting
if(u < RCMin)
    u = RCMin;
elseif(u > RCMax)
    u = RCMax;
end
%dead zone and normalize
 if(u > RCMid + deadZone)
    y = (u-RCMid - deadZone)*k;
 elseif(u < RCMid - deadZone)
     y = (u - RCMid + deadZone)*k;
 else
     y = 0;
 end

 end

== matlab function highgain_with_data_record_param_lowpass/Control System/InputConditioning/deadzone1 ==
  data: u input; y output
function y = fcn(u)
%Function description:
%  Control the range of the remote control input from RCMin to RCMax, and set
%  a dead zone with a dead zone size of ±deadZone,the output y is
%  normalized to 0~1.You can get the RC calibration parameters in QGC.
RCMin = 1065;
RCMax = 1932;
RCMid = (RCMin + RCMax)/2;
deadZoneRate = 0.05;
deadZone = deadZoneRate*(RCMax - RCMin);
k = 1/(RCMax - RCMid - deadZone);
%Limiting
if(u < RCMin)
    u = RCMin;
elseif(u > RCMax)
    u = RCMax;
end
%dead zone and normalize
 if(u > RCMid + deadZone)
    y = (u-RCMid - deadZone)*k;
 elseif(u < RCMid - deadZone)
     y = (u - RCMid + deadZone)*k;
 else
     y = 0;
 end

 end

== matlab function highgain_with_data_record_param_lowpass/Control System/InputConditioning/deadzone2 ==
  data: u input; y output
function y = fcn(u)
%Function description:
%  Control the range of the remote control input from RCMin to RCMax, and set
%  a dead zone with a dead zone size of ±deadZone,the output y is
%  normalized to 0~1.You can get the RC calibration parameters in QGC.
RCMin = 1065;
RCMax = 1932;
RCMid = (RCMin + RCMax)/2;
deadZoneRate = 0.05;
deadZone = deadZoneRate*(RCMax - RCMin);
k = 1/(RCMax - RCMid - deadZone);
%Limiting
if(u < RCMin)
    u = RCMin;
elseif(u > RCMax)
    u = RCMax;
end
%dead zone and normalize
 if(u > RCMid + deadZone)
    y = (u-RCMid - deadZone)*k;
 elseif(u < RCMid - deadZone)
     y = (u - RCMid + deadZone)*k;
 else
     y = 0;
 end

 end

== matlab function highgain_with_data_record_param_lowpass/Control System/Control System1/Subsystem/yaw_lock/MATLAB Function ==
  data: yaw_rate_mode input; yaw_d output; yaw_current input; yaw_d_history input; yaw_d_cal output
function [yaw_d, yaw_d_cal]= UPDATE_YAW(yaw_rate_mode, yaw_current, yaw_d_history)
if(true == yaw_rate_mode) 
    yaw_d_cal = yaw_current;
else
    yaw_d_cal = yaw_d_history;
end

if(true == yaw_rate_mode)
    yaw_d = 0;
else
    yaw_d = yaw_d_cal;
end

end

== matlab function highgain_with_data_record_param_lowpass/Control System/InputConditioning/deadzone3 ==
  data: u input; y output
function y = fcn(u)
%Function description:
%  Control the range of the remote control input from RCMin to RCMax, and set
%  a dead zone with a dead zone size of ±deadZone,the output y is
%  normalized to 0~1.You can get the RC calibration parameters in QGC.
RCMin = 1065;
RCMax = 1932;
RCMid = (RCMin + RCMax)/2;
deadZoneRate = 0.05;
deadZone = deadZoneRate*(RCMax - RCMin);
k = 1/(RCMax - RCMid - deadZone);
%Limiting
if(u < RCMin)
    u = RCMin;
elseif(u > RCMax)
    u = RCMax;
end
%dead zone and normalize
 if(u > RCMid + deadZone)
    y = (u-RCMid - deadZone)*k;
 elseif(u < RCMid - deadZone)
     y = (u - RCMid + deadZone)*k;
 else
     y = 0;
 end

 end

== matlab function highgain_with_data_record_param_lowpass/Control System/Control System1/Subsystem/yaw_lock/MATLAB Function1 ==
  data: rc_yaw input; rate_mode output; rc_thrust_reset input
function rate_mode = yaw_mode_check(rc_yaw, rc_thrust_reset)
    if(rc_yaw ~= 0) || (true == rc_thrust_reset) 
        rate_mode = true;  %%yaw_rate mode
    else
        rate_mode = false;  %%yaw_mode
    end
end

== matlab function highgain_with_data_record_param_lowpass/Control System/Control System1/Subsystem2/MATLAB Function ==
  data: thrust input; f1 input; speed1 output; f2 input; f3 input; f4 input; speed2 output; speed3 output; speed4 output
function [speed1, speed2, speed3, speed4] = force2motor(thrust, f1, f2, f3,f4)
idle_PWM = 1230
scale = 1950 - idle_PWM;
speed1 = (f1 + thrust ) * scale + idle_PWM;
speed2 = (f2 + thrust ) * scale + idle_PWM;
speed3 = (f3 + thrust ) * scale + idle_PWM;
speed4 = (f4 + thrust ) * scale + idle_PWM;
end

== matlab function highgain_with_data_record_param_lowpass/quat2eul ==
  data: q input; phi output; theta output; psi output
function [phi,theta,psi] = quat2eul(q)
% Conversion from Quaternion to Euler angles based on the PX4 Firmware
% v1.6.5 release.
% 
% Quaternion -> DCM -> Euler Angles
% INPUT:
%   q: Quaternion vector of the format: (a + bi + cj + dk)
% OUTPUT:
%   [phi,theta,psi]: Euler angles in radians.
% 
 
    a = q(1);
    b = q(2);
    c = q(3);
    d = q(4);

    aSq = a*a;
    bSq = b*b;
    cSq = c*c;
    dSq = d*d;

    d_pi2 = pi/2;

    % quaternion_to_dcm
    dcm00 = aSq + bSq - cSq - dSq;
    % dcm01 = 2*(b*c - a*d);
    dcm02 = 2*(a*c + b*d);
    dcm10 = 2*(b*c + a*d);
    % dcm11 = aSq - bSq + cSq - dSq;
    dcm12 = 2*(c*d - a*b);
    dcm20 = 2*(b*d - a*c);
    dcm21 = 2*(a*b + c*d);
    dcm22 = aSq - bSq - cSq + dSq;

    % dcm_to_euler
    theta = asin(-dcm20);
    if abs(theta - d_pi2) < 1.0e-3
        phi = single(0.0);
        psi = atan2(dcm12, dcm02);
    elseif abs(theta + d_pi2) < 1.0e-3
        phi = single(0.0);
        psi = atan2(-dcm12, -dcm02);
    else
        phi = atan2(dcm21, dcm22);
        psi = atan2(dcm10, dcm00);
    end

end

== matlab function highgain_with_data_record_param_lowpass/Control System/Control System1/Subsystem2/MATLAB Function2 ==
  data: p input; L output; q input; r input
function L = fcn(p,q,r)
I_xx = 0.0211;I_yy = 0.0211;I_zz = 0.0366;
L = [q * r * (I_yy - I_zz);
     p * r * (I_zz - I_xx);
     p * q * (I_xx - I_yy)];
end
